simulink model "LGS_allFaultsDeselected"  (R2019b)
settings: Solver=FixedStepDiscrete  StartTime=0.0  StopTime=45.0  FixedStep=0.1  RelTol=1e-3
model workspace (MAT data in the model file):
  fipData : object (value not decoded)
  fipName : object (value not decoded)
  stepSize = 0.1
libraries: LibFaultInjectionControls x190, commrandsrc3 x70, simulink x3, LibFailureCondition x1
(part 41 of 41)

== stateflow chart LGS_allFaultsDeselected/FailureConditionObserver/FC2/FC_FC2_output/Chart ==
  state handleIsUp
    en: out = true;
  state handleIsDown
    en: time = int8(149);
    en: out = true;
    du: time = time - 1;
  state gearIsNotDown
    en: out = false;
  state gearIsDown
    en: out = true;
  (default) -> handleIsUp
  gearIsNotDown -> handleIsUp : [(handleUp)]
  gearIsDown -> handleIsUp : [(handleUp)]
  handleIsUp -> handleIsDown : [(~(handleUp))]
  handleIsDown -> handleIsUp [order 1] : [(handleUp)]
  handleIsDown -> gearIsNotDown [order 3] : [(time==0)]
  handleIsDown -> gearIsDown [order 2] : [(gearDown)]
  data: out output boolean; handleUp input boolean; time local int8 [0..150]; gearDown input boolean
